simulink model "FSF_w_disturbance"  (R2020b)
settings: Solver=VariableStepAuto  StartTime=0.0  StopTime=tstop  RelTol=1e-9
undefined symbols (not defined in the file): A, B, d, Dis_Vec, K, x0
settings Model: Creator=domin  LastModifiedBy=domin

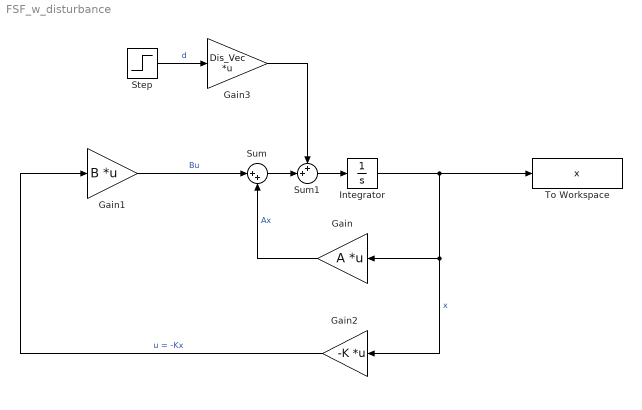
== system FSF_w_disturbance ==
  Gain : Gain  Gain=A  Multiplication=Matrix(K*u)
  Gain1 : Gain  Gain=B  Multiplication=Matrix(K*u)
  Gain2 : Gain  Gain=-K  Multiplication=Matrix(K*u)
  Gain3 : Gain  Gain=Dis_Vec  Multiplication=Matrix(K*u)
  Integrator : Integrator  InitialCondition=x0
  Step : Step  Time=0  After=d  SampleTime=0
  Sum : Sum  Inputs=|++
  Sum1 : Sum  Inputs=++|
  To Workspace : ToWorkspace  VariableName=x  SampleTime=-1
  wires:
  Gain/1 -> Sum/2  "Ax"
  Gain1/1 -> Sum/1  "Bu"
  Integrator/1 -> To Workspace/1, Gain2/1, Gain/1  "x"
  Sum1/1 -> Integrator/1
  Step/1 -> Gain3/1  "d"
  Gain3/1 -> Sum1/1
  Gain2/1 -> Gain1/1  "u = -Kx"
  Sum/1 -> Sum1/2
